simulink model "FanAndPlate_control101"  (R2024a)
settings: Solver=VariableStepAuto  StartTime=0.0  StopTime=Stoptime  FixedStep=0.00001  RelTol=1e-3
PreLoadFcn:
  | run("FanAndPlate_Data_control101.m");
values from neighbouring files (symbols this model uses):
  Ap_P = 0.03    [FanAndPlate_Data_control101.m]    (also in FanAndPlate_model_control101.m)
  Bm_P = 0.014293    [FanAndPlate_Data_control101.m]    (also in FanAndPlate_model_control101.m; OneDofAeroVTOL_Data_control101.m = 0.001; OneDofAeroVTOL_model_control101.m = 0.001)
  Bp_P = 0.028586    [FanAndPlate_Data_control101.m]    (also in FanAndPlate_model_control101.m)
  g_P = 9.81    [FanAndPlate_Data_control101.m]    (also in FanAndPlate_model_control101.m; OneDofAeroVTOL_Data_control101.m; OneDofAeroVTOL_model_control101.m)
  Jm_P = 0.0000536    (= 5.36e-05)    [FanAndPlate_Data_control101.m]    (also in FanAndPlate_model_control101.m; OneDofAeroVTOL_Data_control101.m = 0.000184; OneDofAeroVTOL_model_control101.m = 0.000184)
  Jp_P = 0.00536    [FanAndPlate_Data_control101.m]    (also in FanAndPlate_model_control101.m)
  Kb_P = 0.077    [FanAndPlate_Data_control101.m]    (also in FanAndPlate_model_control101.m; OneDofAeroVTOL_Data_control101.m = 0.0577; OneDofAeroVTOL_model_control101.m = 0.0577)
  Kpl_P = 0.0001    [FanAndPlate_Data_control101.m]    (also in FanAndPlate_model_control101.m; OneDofAeroVTOL_Data_control101.m = 1e-05; OneDofAeroVTOL_model_control101.m = 1e-05)
  Kt_P = 0.077    [FanAndPlate_Data_control101.m]    (also in FanAndPlate_model_control101.m; OneDofAeroVTOL_Data_control101.m = 0.0577; OneDofAeroVTOL_model_control101.m = 0.0577)
  Lm_P = 0.0000177    (= 1.77e-05)    [FanAndPlate_Data_control101.m]    (also in FanAndPlate_model_control101.m; OneDofAeroVTOL_Data_control101.m = 0.00538; OneDofAeroVTOL_model_control101.m = 0.00538)
  lx_P = 0.02    [FanAndPlate_Data_control101.m]    (also in FanAndPlate_model_control101.m)
  mp_P = 0.270    (= 0.27)    [FanAndPlate_Data_control101.m]    (also in FanAndPlate_model_control101.m)
  r_P = 0.06    [FanAndPlate_Data_control101.m]    (also in FanAndPlate_model_control101.m)
  rho_P = 1.293    [FanAndPlate_Data_control101.m]    (also in FanAndPlate_model_control101.m)
  Rm_P = 0.0305    [FanAndPlate_Data_control101.m]    (also in FanAndPlate_model_control101.m; OneDofAeroVTOL_Data_control101.m = 8.4; OneDofAeroVTOL_model_control101.m = 8.4)
undefined symbols (not defined in the file or in its folder): fanspeed, initialcurrent, initialplateangle, initialplatespeed, SampleTime
settings Model: Creator=sword  LastModifiedBy=Anthony Rossiter
settings RTWCC: GPUComputeCapability=3.5
settings ConfigComp: CovBoundaryAbsTol=1.0e-5

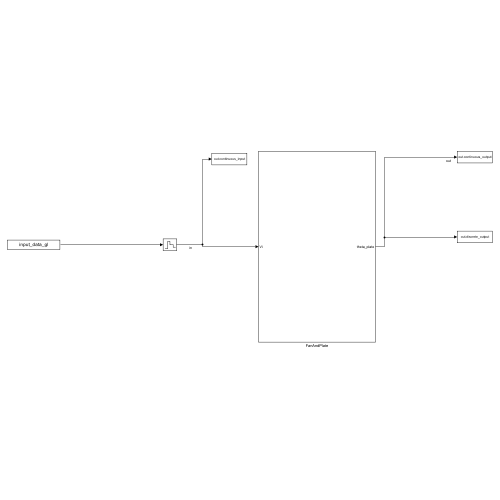
[thumbnail: Simulink's stored preview of the top-level diagram]
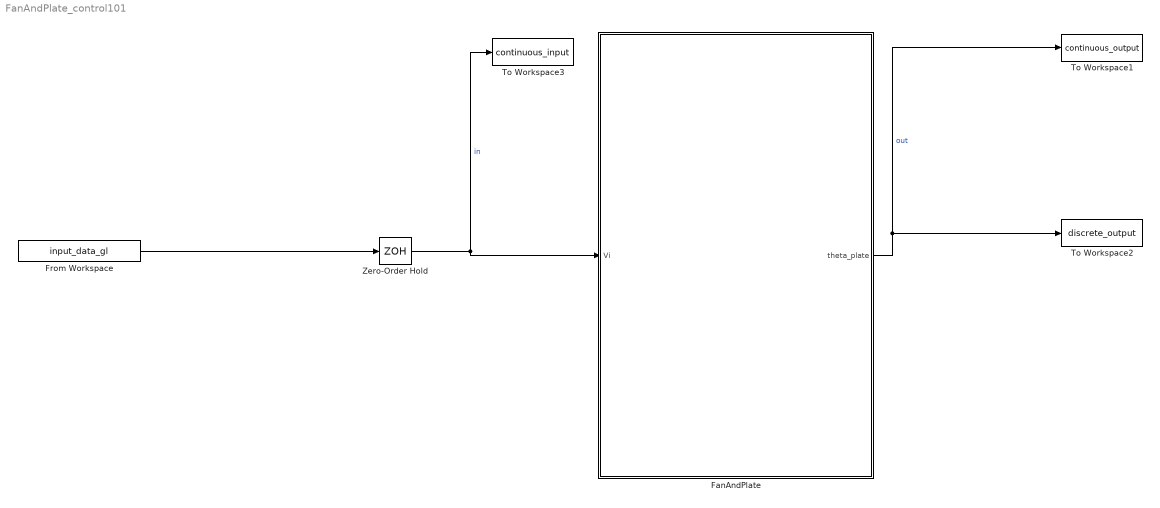
== system FanAndPlate_control101 ==
  FanAndPlate : Subsystem
  From Workspace : FromWorkspace  VariableName=input_data_gl  SampleTime=SampleTime
  To Workspace1 : ToWorkspace  VariableName=continuous_output  SaveFormat=Structure With Time  SampleTime=0.0001
  To Workspace2 : ToWorkspace  VariableName=discrete_output  SaveFormat=Structure With Time  SampleTime=SampleTime
  To Workspace3 : ToWorkspace  VariableName=continuous_input  SaveFormat=Structure With Time  SampleTime=-1
  Zero-Order Hold : ZeroOrderHold  SampleTime=SampleTime
  wires:
  FanAndPlate/1(theta_plate) -> To Workspace1/1, To Workspace2/1  "out"
  From Workspace/1 -> Zero-Order Hold/1
  Zero-Order Hold/1 -> FanAndPlate/1(Vi), To Workspace3/1  "in"

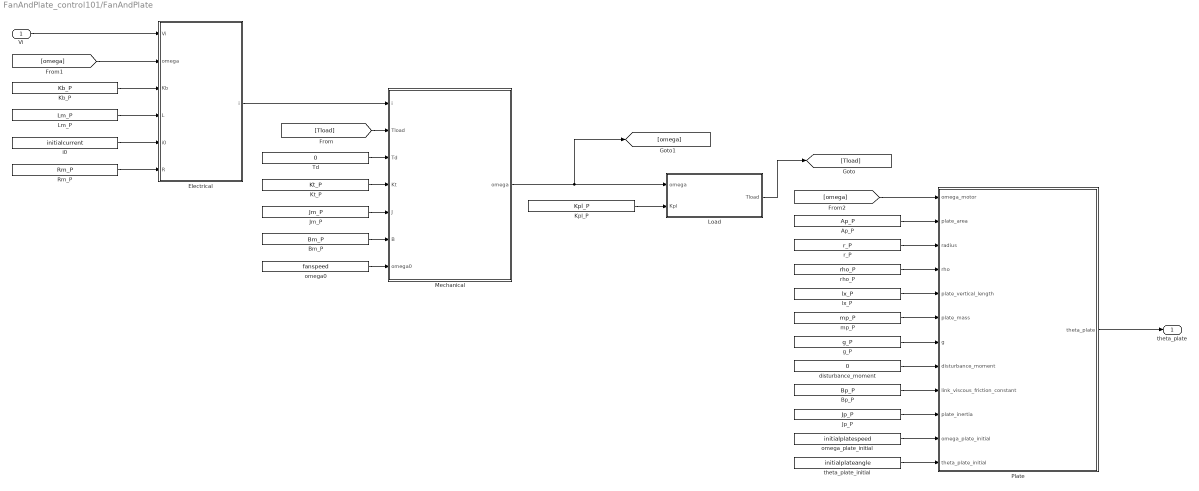
== system FanAndPlate_control101/FanAndPlate ==
  Vi : Inport
  Ap_P : Constant  Value=Ap_P  OutDataTypeStr=Inherit: Inherit via back propagation  SampleTime=-1
  Bm_P : Constant  Value=Bm_P  OutDataTypeStr=Inherit: Inherit via back propagation  SampleTime=-1
  Bp_P : Constant  Value=Bp_P  OutDataTypeStr=Inherit: Inherit via back propagation  SampleTime=-1
  Electrical : Subsystem
  Jm_P : Constant  Value=Jm_P  OutDataTypeStr=Inherit: Inherit via back propagation  SampleTime=-1
  Jp_P : Constant  Value=Jp_P  OutDataTypeStr=Inherit: Inherit via back propagation  SampleTime=-1
  Kb_P : Constant  Value=Kb_P  OutDataTypeStr=Inherit: Inherit via back propagation  SampleTime=-1
  Kpl_P : Constant  Value=Kpl_P  OutDataTypeStr=Inherit: Inherit via back propagation  SampleTime=-1
  Kt_P : Constant  Value=Kt_P  OutDataTypeStr=Inherit: Inherit via back propagation  SampleTime=-1
  Lm_P : Constant  Value=Lm_P  OutDataTypeStr=Inherit: Inherit via back propagation  SampleTime=-1
  Load : Subsystem
  Mechanical : Subsystem
  Plate : Subsystem
  Rm_P : Constant  Value=Rm_P  OutDataTypeStr=Inherit: Inherit via back propagation  SampleTime=-1
  Td : Constant  Value=0  OutDataTypeStr=Inherit: Inherit via back propagation  SampleTime=-1
  disturbance_moment : Constant  Value=0  OutDataTypeStr=Inherit: Inherit via back propagation  SampleTime=-1
  g_P : Constant  Value=g_P  OutDataTypeStr=Inherit: Inherit via back propagation  SampleTime=-1
  i0 : Constant  Value=initialcurrent  OutDataTypeStr=Inherit: Inherit via back propagation  SampleTime=-1
  lx_P : Constant  Value=lx_P  OutDataTypeStr=Inherit: Inherit via back propagation  SampleTime=-1
  mp_P : Constant  Value=mp_P  OutDataTypeStr=Inherit: Inherit via back propagation  SampleTime=-1
  omega0 : Constant  Value=fanspeed  OutDataTypeStr=Inherit: Inherit via back propagation  SampleTime=-1
  omega_plate_initial : Constant  Value=initialplatespeed  OutDataTypeStr=Inherit: Inherit via back propagation  SampleTime=-1
  r_P : Constant  Value=r_P  OutDataTypeStr=Inherit: Inherit via back propagation  SampleTime=-1
  rho_P : Constant  Value=rho_P  OutDataTypeStr=Inherit: Inherit via back propagation  SampleTime=-1
  theta_plate_initial : Constant  Value=initialplateangle  OutDataTypeStr=Inherit: Inherit via back propagation  SampleTime=-1
  theta_plate : Outport  VectorParamsAs1DForOutWhenUnconnected=off
  wires:
  g_P/1 -> Plate/7(g)
  theta_plate_initial/1 -> Plate/12(theta_plate_initial)
  Plate/1(theta_plate) -> theta_plate/1
  Bp_P/1 -> Plate/9(link_viscous_friction_constant)
  mp_P/1 -> Plate/6(plate_mass)
  Jp_P/1 -> Plate/10(plate_inertia)
  Ap_P/1 -> Plate/2(plate_area)
  disturbance_moment/1 -> Plate/8(disturbance_moment)
  lx_P/1 -> Plate/5(plate_vertical_length)
  omega_plate_initial/1 -> Plate/11(omega_plate_initial)
  Electrical/1(i) -> Mechanical/1(i)
  Mechanical/1(omega) -> [omega], Load/1(omega)
  Vi/1 -> Electrical/1(Vi)
  Load/1(Tload) -> [Tload]
  [Tload] -> Mechanical/2(Tload)
  Td/1 -> Mechanical/3(Td)
  [omega] -> Electrical/2(omega)
  Kb_P/1 -> Electrical/3(Kb)
  i0/1 -> Electrical/5(i0)
  Lm_P/1 -> Electrical/4(L)
  Rm_P/1 -> Electrical/6(R)
  Kpl_P/1 -> Load/2(Kpl)
  Kt_P/1 -> Mechanical/4(Kt)
  Jm_P/1 -> Mechanical/5(J)
  Bm_P/1 -> Mechanical/6(B)
  omega0/1 -> Mechanical/7(omega0)
  r_P/1 -> Plate/3(radius)
  rho_P/1 -> Plate/4(rho)
  [omega] -> Plate/1(omega_motor)

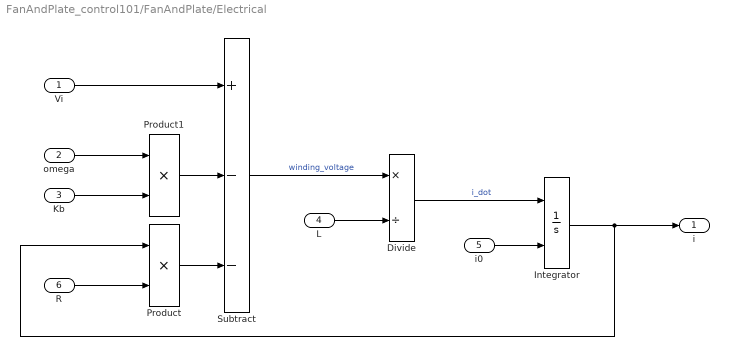
== system FanAndPlate_control101/FanAndPlate/Electrical ==
  Vi : Inport
  omega : Inport  Port=2
  Kb : Inport  Port=3
  L : Inport  Port=4
  i0 : Inport  Port=5
  R : Inport  Port=6
  Divide : Product  Inputs=*/  RndMeth=Zero  SaturateOnIntegerOverflow=on  OutDataTypeStr=Inherit: Same as first input
  Integrator : Integrator  InitialConditionSource=external  ContinuousStateAttributes='current'
  Product : Product  InputSameDT=on  RndMeth=Zero  SaturateOnIntegerOverflow=on  OutDataTypeStr=Inherit: Same as first input
  Product1 : Product  InputSameDT=on  RndMeth=Zero  SaturateOnIntegerOverflow=on  OutDataTypeStr=Inherit: Same as first input
  Subtract : Sum  Inputs=+--  InputSameDT=on  RndMeth=Zero  SaturateOnIntegerOverflow=on
  i : Outport
  wires:
  Kb/1 -> Product1/2
  omega/1 -> Product1/1
  Product1/1 -> Subtract/2
  R/1 -> Product/2
  Product/1 -> Subtract/3
  Integrator/1 -> i/1, Product/1
  i0/1 -> Integrator/2
  Divide/1 -> Integrator/1  "i_dot"
  L/1 -> Divide/2
  Subtract/1 -> Divide/1  "winding_voltage"
  Vi/1 -> Subtract/1

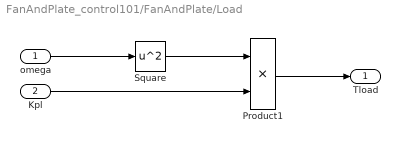
== system FanAndPlate_control101/FanAndPlate/Load ==
  omega : Inport
  Kpl : Inport  Port=2
  Product1 : Product  InputSameDT=on  RndMeth=Zero  SaturateOnIntegerOverflow=on  OutDataTypeStr=Inherit: Same as first input
  Square : Math  Operator=square
  Tload : Outport
  wires:
  Product1/1 -> Tload/1
  Kpl/1 -> Product1/2
  Square/1 -> Product1/1
  omega/1 -> Square/1

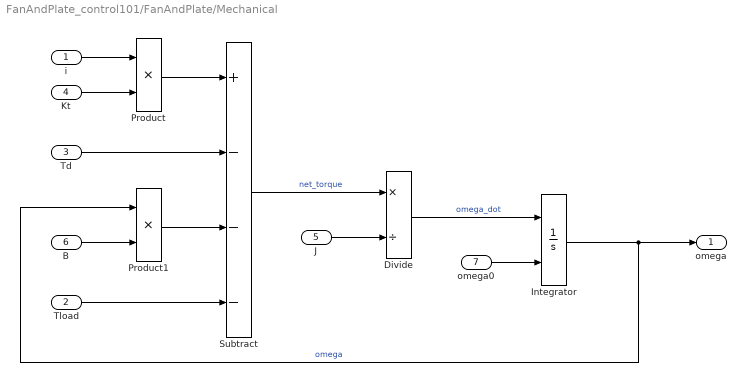
== system FanAndPlate_control101/FanAndPlate/Mechanical ==
  i : Inport
  Tload : Inport  Port=2
  Td : Inport  Port=3
  Kt : Inport  Port=4
  J : Inport  Port=5
  B : Inport  Port=6
  omega0 : Inport  Port=7
  Divide : Product  Inputs=*/  RndMeth=Zero  SaturateOnIntegerOverflow=on  OutDataTypeStr=Inherit: Same as first input
  Integrator : Integrator  InitialConditionSource=external  ContinuousStateAttributes='motor_speed'
  Product : Product  InputSameDT=on  RndMeth=Zero  SaturateOnIntegerOverflow=on  OutDataTypeStr=Inherit: Same as first input
  Product1 : Product  InputSameDT=on  RndMeth=Zero  SaturateOnIntegerOverflow=on  OutDataTypeStr=Inherit: Same as first input
  Subtract : Sum  Inputs=+---  InputSameDT=on  RndMeth=Zero  SaturateOnIntegerOverflow=on
  omega : Outport
  wires:
  Tload/1 -> Subtract/4
  Td/1 -> Subtract/2
  B/1 -> Product1/2
  Product1/1 -> Subtract/3
  Integrator/1 -> Product1/1, omega/1  "omega"
  Subtract/1 -> Divide/1  "net_torque"
  Divide/1 -> Integrator/1  "omega_dot"
  omega0/1 -> Integrator/2
  J/1 -> Divide/2
  Product/1 -> Subtract/1
  Kt/1 -> Product/2
  i/1 -> Product/1

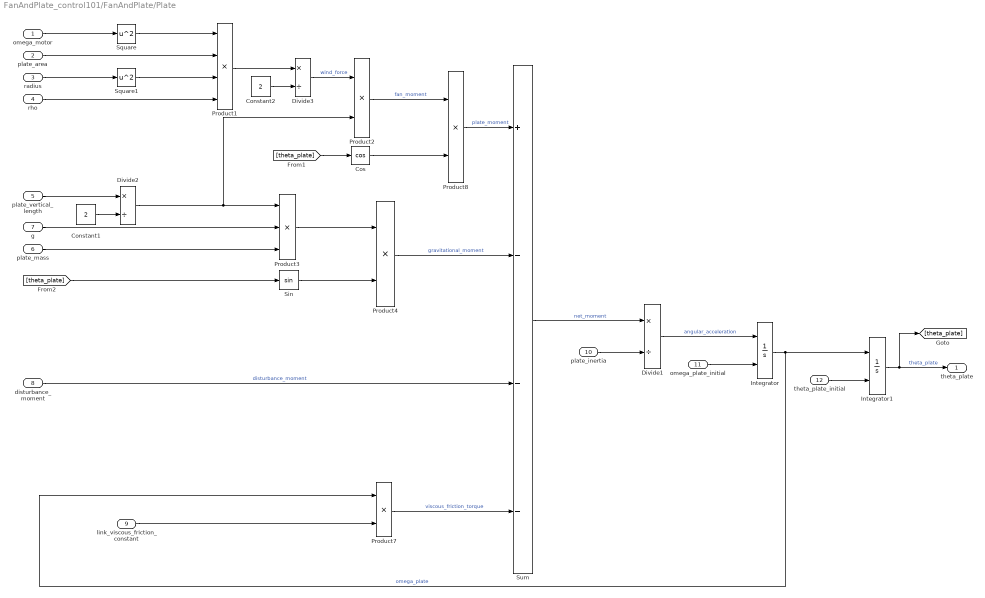
== system FanAndPlate_control101/FanAndPlate/Plate ==
  omega_motor : Inport
  plate_area : Inport  Port=2
  radius : Inport  Port=3
  rho : Inport  Port=4
  plate_vertical_length : Inport  Port=5
  plate_mass : Inport  Port=6
  g : Inport  Port=7
  disturbance_moment : Inport  Port=8
  link_viscous_friction_constant : Inport  Port=9
  plate_inertia : Inport  Port=10
  omega_plate_initial : Inport  Port=11
  theta_plate_initial : Inport  Port=12
  Constant1 : Constant  Value=2  OutDataTypeStr=Inherit: Inherit via back propagation  SampleTime=-1
  Constant2 : Constant  Value=2  OutDataTypeStr=Inherit: Inherit via back propagation  SampleTime=-1
  Cos : Trigonometry  Operator=cos
  Divide1 : Product  Inputs=*/  RndMeth=Zero  SaturateOnIntegerOverflow=on  OutDataTypeStr=Inherit: Same as first input
  Divide2 : Product  Inputs=*/  RndMeth=Zero  SaturateOnIntegerOverflow=on  OutDataTypeStr=Inherit: Same as first input
  Divide3 : Product  Inputs=*/  RndMeth=Zero  SaturateOnIntegerOverflow=on  OutDataTypeStr=Inherit: Same as first input
  Integrator : Integrator  InitialConditionSource=external  ContinuousStateAttributes='omega_plate'
  Integrator1 : Integrator  InitialConditionSource=external  ContinuousStateAttributes='theta_plate'
  Product1 : Product  Inputs=4  InputSameDT=on  RndMeth=Zero  SaturateOnIntegerOverflow=on  OutDataTypeStr=Inherit: Same as first input
  Product{2,4,7..8} (4 alike) : Product  InputSameDT=on  RndMeth=Zero  SaturateOnIntegerOverflow=on  OutDataTypeStr=Inherit: Same as first input
  Product3 : Product  Inputs=3  InputSameDT=on  RndMeth=Zero  SaturateOnIntegerOverflow=on  OutDataTypeStr=Inherit: Same as first input
  Sin : Trigonometry
  Square : Math  Operator=square
  Square1 : Math  Operator=square
  Sum : Sum  Inputs=+---  OutDataTypeStr=Inherit: Inherit via back propagation  InputSameDT=on  RndMeth=Zero  SaturateOnIntegerOverflow=on
  theta_plate : Outport
  wires:
  [theta_plate] -> Sin/1
  plate_mass/1 -> Product3/3
  g/1 -> Product3/2
  [theta_plate] -> Cos/1
  Product8/1 -> Sum/1  "plate_moment"
  Cos/1 -> Product8/2
  Product2/1 -> Product8/1  "fan_moment"
  Constant1/1 -> Divide2/2
  Square/1 -> Product1/1
  Divide3/1 -> Product2/1  "wind_force"
  Product3/1 -> Product4/1
  Sin/1 -> Product4/2
  Product4/1 -> Sum/2  "gravitational_moment"
  disturbance_moment/1 -> Sum/3  "disturbance_moment"
  Product7/1 -> Sum/4  "viscous_friction_torque"
  link_viscous_friction_constant/1 -> Product7/2
  Sum/1 -> Divide1/1  "net_moment"
  plate_inertia/1 -> Divide1/2
  Divide1/1 -> Integrator/1  "angular_acceleration"
  omega_plate_initial/1 -> Integrator/2
  Integrator1/1 -> [theta_plate], theta_plate/1  "theta_plate"
  Integrator/1 -> Integrator1/1, Product7/1  "omega_plate"
  theta_plate_initial/1 -> Integrator1/2
  omega_motor/1 -> Square/1
  radius/1 -> Square1/1
  plate_area/1 -> Product1/2
  Square1/1 -> Product1/3
  rho/1 -> Product1/4
  plate_vertical_length/1 -> Divide2/1
  Constant2/1 -> Divide3/2
  Product1/1 -> Divide3/1
  Divide2/1 -> Product2/2, Product3/1
